simulink model "PM"  (R2018a)
settings: Solver=ode4  StartTime=0.0  StopTime=2  MaxStep=0.2  RelTol=1e-4
libraries: powerlib x20, simulink x13
settings Model: Creator=user  LastModifiedBy=user
settings CodeAppCC: StateflowObjectComments=on

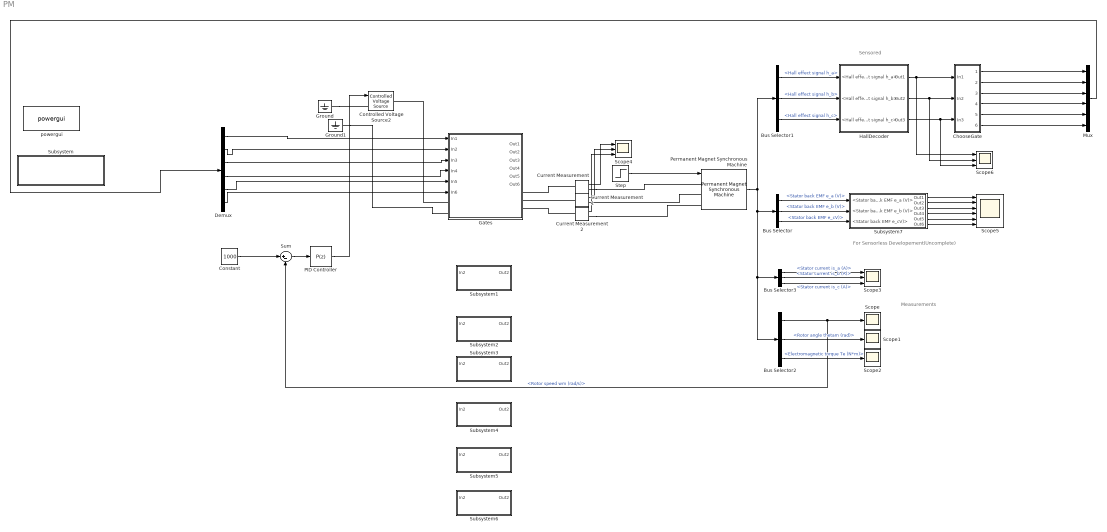
== system PM ==
  note: Measurements
  note: For Sensorless Developement(Uncomplete)
  note: Sensored
  Bus Selector : BusSelector  OutputSignals=Stator back EMF e_a (V),Stator back EMF e_b (V),Stator back EMF e_cV)
  Bus Selector1 : BusSelector  OutputSignals=Hall effect signal h_a,Hall effect signal h_b,Hall effect signal h_c
  Bus Selector2 : BusSelector  OutputSignals=Rotor speed wm (rad/s),Rotor angle thetam (rad),Electromagnetic torque Te (N*m)
  Bus Selector3 : BusSelector  OutputSignals=Stator current is_a (A),Stator current is_b (A),Stator current is_c (A)
  ChooseGate : Subsystem
  Constant : Constant  Value=1000
  Controlled Voltage Source2 : powerlib/Electrical Sources/Controlled Voltage Source  Initialize=on  Source_Type=AC  Amplitude=50  Phase=0  Frequency=0  Measurements=None
  Current Measurement : powerlib/Measurements/Current Measurement  PhasorSimulation=off  OutputType=Complex  PSBequivalent=0
  Current Measurement1 : powerlib/Measurements/Current Measurement  PhasorSimulation=off  OutputType=Complex  PSBequivalent=0
  Current Measurement2 : powerlib/Measurements/Current Measurement  PhasorSimulation=off  OutputType=Complex  PSBequivalent=0
  Demux : Demux  Outputs=6
  Gates : Subsystem
  Ground : powerlib/Elements/Ground  LConnTagsString=a
  Ground1 : powerlib/Elements/Ground  LConnTagsString=a
  HallDecoder : Subsystem
  Mux : Mux  Inputs=6
  PID Controller : simulink/Continuous/PID Controller  Controller=P  TimeDomain=Discrete-time  SampleTime=-1  IntegratorMethod=Forward Euler  FilterMethod=Forward Euler  Form=Parallel  UseFilter=on  ControllerParametersSource=internal  P=15.2669895958737  I=1  D=0  N=100  InitialConditionSource=internal  InitialConditionForIntegrator=0  InitialConditionForFilter=0  ExternalReset=none  LimitOutput=off  UpperSaturationLimit=inf  LowerSaturationLimit=-inf  LinearizeAsGain=on  AntiWindupMode=none  Kb=1  TrackingMode=off  Kt=1  PParamMin=[]  PParamMax=[]  IParamMin=[]  IParamMax=[]  DParamMin=[]  DParamMax=[]  NParamMin=[]  NParamMax=[]  KbParamMin=[]  KbParamMax=[]  KtParamMin=[]  KtParamMax=[]  POutMin=[]  POutMax=[]  IOutMin=[]  IOutMax=[]  DOutMin=[]  DOutMax=[]  NOutMin=[]  NOutMax=[]  KbOutMin=[]  KbOutMax=[]  KtOutMin=[]  KtOutMax=[]  IntegratorOutMin=[]  IntegratorOutMax=[]  FilterOutMin=[]  FilterOutMax=[]  SumOutMin=[]  SumOutMax=[]  SumI1OutMin=[]  SumI1OutMax=[]  SumI2OutMin=[]  SumI2OutMax=[]  SumI3OutMin=[]  SumI3OutMax=[]  SumDOutMin=[]  SumDOutMax=[]  SaturationOutMin=[]  SaturationOutMax=[]  IntegratorContinuousStateAttributes=''  IntegratorStateMustResolveToSignalObject=off  IntegratorRTWStateStorageClass=Auto  FilterContinuousStateAttributes=''  FilterStateMustResolveToSignalObject=off  FilterRTWStateStorageClass=Auto  DifferentiatorICPrevScaledInput=0  DifferentiatorOutMin=[]  DifferentiatorOutMax=[]  FilterDiffOutCoefMin=[]  FilterDiffOutCoefMax=[]  SumDenOutMin=[]  SumDenOutMax=[]  SumNumOutMin=[]  SumNumOutMax=[]  ReciprocalOutMin=[]  ReciprocalOutMax=[]  DivideOutMin=[]  DivideOutMax=[]  TunerSelectOption=Transfer Function Based (PID Tuner App)
  Permanent Magnet Synchronous Machine : powerlib/Machines/Permanent Magnet Synchronous Machine  NbPhases=3  FluxDistribution=Trapezoidal  RotorType=Round  MechanicalLoad=Torque Tm  PresetModel=No  ShowDetailedParameters=on  MeasurementBus=off  Resistance=2.8750  Inductance=8.5e-3  dqInductances=[8.5e-3, 8.5e-3]  La=0.000835  MachineConstant=Flux linkage established by magnets (V.s)  Flux=0.175  VoltageCst=146.6077  TorqueCst=1.4  Flat=120  Mechanical=[ 0.8e-3, 1e-3 4]  PolePairs=4  InitialConditions=[0,0, 0,0]  InitialConditions5ph=[0 0 0 0 0 0]  TsPowergui=0  TsBlock=-1  RefAngle=90 degrees behind phase A axis (modified Park)
      settings: SourceProductName=Simscape Power Systems
  Scope : Scope
  Scope1 : Scope
  Scope2 : Scope
  Scope3 : Scope  NumInputPorts=3
  Scope4 : Scope  NumInputPorts=3
  Scope5 : Scope  NumInputPorts=6
  Scope6 : Scope  NumInputPorts=3
  Step : Step  Time=0.01  After=2  SampleTime=0
  Subsystem : Subsystem
      settings: OpenFcn=open_system('power_new_palette')
      mask Display: disp(sprintf('Open Simscape Power Systems\n(Specialized Technology)\nPalette Library'));
  Subsystem1 : Subsystem
  Subsystem2 : Subsystem
  Subsystem3 : Subsystem
  Subsystem4 : Subsystem
  Subsystem5 : Subsystem
  Subsystem6 : Subsystem
  Subsystem7 : Subsystem
  Sum : Sum  Inputs=|+-
  powergui : powerlib/powergui  Priority=1  SimulationMode=Discrete  SampleTime=5e-6  frequency=60  Iterations=50  frequencyindice=0  Pbase=100e6  ErrMax=1e-4  UnitsV=kV  UnitsW=MW  buscounter=0  FunctionMessages=off  echomessages=off  EnableUseOfTLC=off  CurrentSourceSwitches=off  DisableSnubberDevices=off  DisableRonSwitches=off  DisableVfSwitches=off  DisplayEquations=off  SolverType=Tustin/Backward Euler (TBE)  Interpol=off  ExternalGateDelay=off  methode=off  Ts=100  x0status=blocks  SPID=on  SwTol=0  HookPort=off  RestoreLinks=warning  ResistiveCurrentMeasurement=off  Frange=[0:2:500]  Ylog=off  Xlog=on  ShowGrid=off  save=off  variable=ZData  structure=0  ZoomFFT=off  StartTime=0.0  cycles=1  DisplayStyle=1  fundamental=60  FreqAxis=off  MaxFrequency=1000  frequencyindicesteady=1  RmsSteady=1  display=off
  wires:
  Permanent Magnet Synchronous Machine/1 -> Bus Selector2/1, Bus Selector3/1, Bus Selector/1, Bus Selector1/1
  Bus Selector1/1 -> HallDecoder/1(<Hall effect signal h_a>)  "<Hall effect signal h_a>"
  Bus Selector1/2 -> HallDecoder/2(<Hall effect signal h_b>)  "<Hall effect signal h_b>"
  Bus Selector1/3 -> HallDecoder/3(<Hall effect signal h_c>)  "<Hall effect signal h_c>"
  HallDecoder/3(Out3) -> Scope6/3, ChooseGate/3(In3)
  HallDecoder/2(Out2) -> Scope6/2, ChooseGate/2(In2)
  HallDecoder/1(Out1) -> Scope6/1, ChooseGate/1(In1)
  Mux/1 -> Demux/1
  Bus Selector2/1 -> Sum/2, Scope/1  "<Rotor speed wm (rad/s)>"
  Bus Selector2/2 -> Scope1/1  "<Rotor angle thetam (rad)>"
  Bus Selector2/3 -> Scope2/1  "<Electromagnetic torque Te (N*m)>"
  Bus Selector3/2 -> Scope3/2  "<Stator current is_b (A)>"
  Bus Selector3/3 -> Scope3/3  "<Stator current is_c (A)>"
  Bus Selector3/1 -> Scope3/1  "<Stator current is_a (A)>"
  Current Measurement/1 -> Scope4/1
  Current Measurement2/1 -> Scope4/3
  Step/1 -> Permanent Magnet Synchronous Machine/1
  Current Measurement1/1 -> Scope4/2
  ChooseGate/1(Out1) -> Mux/1
  ChooseGate/2(Out2) -> Mux/2
  ChooseGate/3(Out3) -> Mux/3
  ChooseGate/4(Out4) -> Mux/4
  ChooseGate/5(Out5) -> Mux/5
  ChooseGate/6(Out6) -> Mux/6
  Bus Selector/1 -> Subsystem7/1(<Stator back EMF e_a (V)>)  "<Stator back EMF e_a (V)>"
  Bus Selector/2 -> Subsystem7/2(<Stator back EMF e_b (V)>)  "<Stator back EMF e_b (V)>"
  Bus Selector/3 -> Subsystem7/3(<Stator back EMF e_cV)>)  "<Stator back EMF e_cV)>"
  Subsystem7/1(Out1) -> Scope5/1
  Subsystem7/2(Out2) -> Scope5/2
  Subsystem7/3(Out3) -> Scope5/3
  Subsystem7/4(Out4) -> Scope5/4
  Subsystem7/5(Out5) -> Scope5/5
  Subsystem7/6(Out6) -> Scope5/6
  Demux/1 -> Gates/1(In1)
  Demux/2 -> Gates/2(In2)
  Demux/3 -> Gates/3(In3)
  Demux/4 -> Gates/4(In4)
  Demux/5 -> Gates/5(In5)
  Demux/6 -> Gates/6(In6)
  PID Controller/1 -> Controlled Voltage Source2/1
  Constant/1 -> Sum/1
  Sum/1 -> PID Controller/1
  connections:
  Ground/LConn1 -- Controlled Voltage Source2/LConn1
  Current Measurement/RConn1 -- Permanent Magnet Synchronous Machine/LConn1
  Permanent Magnet Synchronous Machine/LConn2 -- Current Measurement1/RConn1
  Current Measurement2/RConn1 -- Permanent Magnet Synchronous Machine/LConn3
  Current Measurement/LConn1 -- Gates/RConn1
  Gates/LConn1 -- Controlled Voltage Source2/RConn1
  Current Measurement1/LConn1 -- Gates/RConn2
  Ground1/LConn1 -- Gates/LConn2
  Current Measurement2/LConn1 -- Gates/RConn3

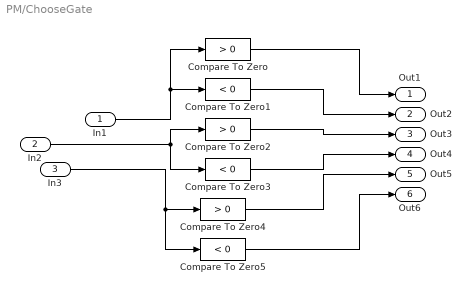
== system PM/ChooseGate ==
  In1 : Inport
  In2 : Inport  Port=2
  In3 : Inport  Port=3
  Compare To Zero : simulink/Logic and Bit Operations/Compare To Zero  relop=>  OutDataTypeStr=boolean  ZeroCross=off
  Compare To Zero1 : simulink/Logic and Bit Operations/Compare To Zero  relop=<  OutDataTypeStr=boolean  ZeroCross=off
  Compare To Zero2 : simulink/Logic and Bit Operations/Compare To Zero  relop=>  OutDataTypeStr=boolean  ZeroCross=off
  Compare To Zero3 : simulink/Logic and Bit Operations/Compare To Zero  relop=<  OutDataTypeStr=boolean  ZeroCross=off
  Compare To Zero4 : simulink/Logic and Bit Operations/Compare To Zero  relop=>  OutDataTypeStr=boolean  ZeroCross=off
  Compare To Zero5 : simulink/Logic and Bit Operations/Compare To Zero  relop=<  OutDataTypeStr=boolean  ZeroCross=off
  Out1 : Outport
  Out2 : Outport  Port=2
  Out3 : Outport  Port=3
  Out4 : Outport  Port=4
  Out5 : Outport  Port=5
  Out6 : Outport  Port=6
  wires:
  In3/1 -> Compare To Zero4/1, Compare To Zero5/1
  Compare To Zero/1 -> Out1/1
  In1/1 -> Compare To Zero/1, Compare To Zero1/1
  Compare To Zero1/1 -> Out2/1
  In2/1 -> Compare To Zero2/1, Compare To Zero3/1
  Compare To Zero5/1 -> Out6/1
  Compare To Zero4/1 -> Out5/1
  Compare To Zero3/1 -> Out4/1
  Compare To Zero2/1 -> Out3/1

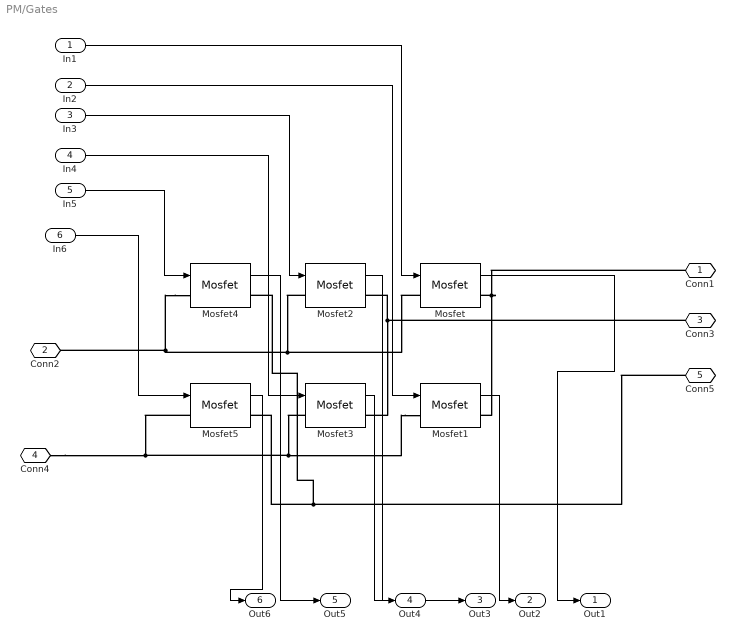
== system PM/Gates ==
  In1 : Inport
  In2 : Inport  Port=2
  In3 : Inport  Port=3
  In4 : Inport  Port=4
  In5 : Inport  Port=5
  In6 : Inport  Port=6
  Mosfet{,1..5} (6 alike) : powerlib/Power Electronics/Mosfet  Ron=0.1  Lon=0  Rd=0.01  Vfd=0  IC=0  Rs=1e5  Cs=inf  Measurements=on
  Conn1 : PMIOPort  Side=Right
  Conn2 : PMIOPort  Port=2  Side=Left
  Conn3 : PMIOPort  Port=3  Side=Right
  Conn4 : PMIOPort  Port=4  Side=Left
  Conn5 : PMIOPort  Port=5  Side=Right
  Out1 : Outport
  Out2 : Outport  Port=2
  Out3 : Outport  Port=3
  Out4 : Outport  Port=4
  Out5 : Outport  Port=5
  Out6 : Outport  Port=6
  wires:
  Mosfet/1 -> Out1/1
  In2/1 -> Mosfet1/1
  Mosfet1/1 -> Out2/1
  In3/1 -> Mosfet2/1
  Mosfet5/1 -> Out6/1
  In1/1 -> Mosfet/1
  Mosfet4/1 -> Out5/1
  Mosfet2/1 -> Out3/1
  Mosfet3/1 -> Out4/1
  In4/1 -> Mosfet3/1
  In5/1 -> Mosfet4/1
  In6/1 -> Mosfet5/1
  connections:
  Conn3/RConn1 -- Mosfet3/RConn1 -- Mosfet2/RConn1
  Conn5/RConn1 -- Mosfet4/RConn1 -- Mosfet5/RConn1
  Mosfet1/LConn1 -- Mosfet3/LConn1 -- Mosfet5/LConn1 -- Conn4/RConn1
  Mosfet4/LConn1 -- Mosfet2/LConn1 -- Mosfet/LConn1 -- Conn2/RConn1
  Mosfet/RConn1 -- Conn1/RConn1 -- Mosfet1/RConn1

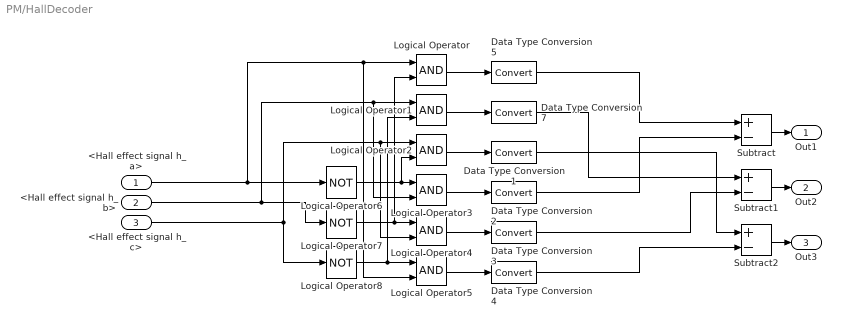
== system PM/HallDecoder ==
  <Hall effect signal h_a> : Inport
  <Hall effect signal h_b> : Inport  Port=2
  <Hall effect signal h_c> : Inport  Port=3
  Data Type Conversion{1..5,7} (6 alike) : DataTypeConversion
  Logical Operator{,1..5} (6 alike) : Logic  AllPortsSameDT=off  OutDataTypeStr=boolean
  Logical Operator6 : Logic  Operator=NOT  AllPortsSameDT=off  OutDataTypeStr=boolean
  Logical Operator7 : Logic  Operator=NOT  AllPortsSameDT=off  OutDataTypeStr=boolean
  Logical Operator8 : Logic  Operator=NOT  AllPortsSameDT=off  OutDataTypeStr=boolean
  Subtract : Sum  Inputs=+-
  Subtract1 : Sum  Inputs=+-
  Subtract2 : Sum  Inputs=+-
  Out1 : Outport
  Out2 : Outport  Port=2
  Out3 : Outport  Port=3
  wires:
  <Hall effect signal h_a>/1 -> Logical Operator6/1, Logical Operator5/2, Logical Operator/1
  Logical Operator6/1 -> Logical Operator2/2, Logical Operator3/1
  <Hall effect signal h_b>/1 -> Logical Operator7/1, Logical Operator1/1, Logical Operator3/2
  <Hall effect signal h_c>/1 -> Logical Operator8/1, Logical Operator4/2, Logical Operator2/1
  Logical Operator8/1 -> Logical Operator1/2, Logical Operator5/1
  Logical Operator7/1 -> Logical Operator4/1, Logical Operator/2
  Subtract2/1 -> Out3/1
  Subtract1/1 -> Out2/1
  Subtract/1 -> Out1/1
  Logical Operator/1 -> Data Type Conversion5/1
  Logical Operator1/1 -> Data Type Conversion7/1
  Logical Operator2/1 -> Data Type Conversion1/1
  Logical Operator3/1 -> Data Type Conversion2/1
  Logical Operator4/1 -> Data Type Conversion3/1
  Logical Operator5/1 -> Data Type Conversion4/1
  Data Type Conversion5/1 -> Subtract/1
  Data Type Conversion2/1 -> Subtract/2
  Data Type Conversion7/1 -> Subtract1/1
  Data Type Conversion3/1 -> Subtract1/2
  Data Type Conversion1/1 -> Subtract2/1
  Data Type Conversion4/1 -> Subtract2/2

== system PM/Subsystem ==

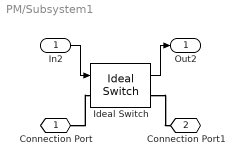
== system PM/Subsystem1 ==
  In2 : Inport
  Ideal Switch : powerlib/Power Electronics/Ideal Switch  Ron=0.001  Lon=0  IC=1  Rs=1e5  Cs=inf  Measurements=on
  Connection Port : PMIOPort  Side=Left
  Connection Port1 : PMIOPort  Port=2  Side=Right
  Out2 : Outport
  wires:
  In2/1 -> Ideal Switch/1
  Ideal Switch/1 -> Out2/1
  connections:
  Ideal Switch/RConn1 -- Connection Port1/RConn1
  Connection Port/RConn1 -- Ideal Switch/LConn1

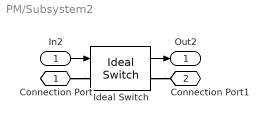
== system PM/Subsystem2 ==
  In2 : Inport
  Ideal Switch : powerlib/Power Electronics/Ideal Switch  Ron=0.001  Lon=0  IC=1  Rs=1e5  Cs=inf  Measurements=on
  Connection Port : PMIOPort  Side=Left
  Connection Port1 : PMIOPort  Port=2  Side=Right
  Out2 : Outport
  wires:
  In2/1 -> Ideal Switch/1
  Ideal Switch/1 -> Out2/1
  connections:
  Ideal Switch/RConn1 -- Connection Port1/RConn1
  Connection Port/RConn1 -- Ideal Switch/LConn1

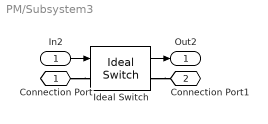
== system PM/Subsystem3 ==
  In2 : Inport
  Ideal Switch : powerlib/Power Electronics/Ideal Switch  Ron=0.001  Lon=0  IC=1  Rs=1e5  Cs=inf  Measurements=on
  Connection Port : PMIOPort  Side=Left
  Connection Port1 : PMIOPort  Port=2  Side=Right
  Out2 : Outport
  wires:
  In2/1 -> Ideal Switch/1
  Ideal Switch/1 -> Out2/1
  connections:
  Ideal Switch/RConn1 -- Connection Port1/RConn1
  Connection Port/RConn1 -- Ideal Switch/LConn1

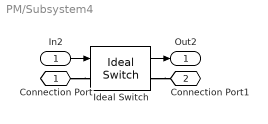
== system PM/Subsystem4 ==
  In2 : Inport
  Ideal Switch : powerlib/Power Electronics/Ideal Switch  Ron=0.001  Lon=0  IC=1  Rs=1e5  Cs=inf  Measurements=on
  Connection Port : PMIOPort  Side=Left
  Connection Port1 : PMIOPort  Port=2  Side=Right
  Out2 : Outport
  wires:
  In2/1 -> Ideal Switch/1
  Ideal Switch/1 -> Out2/1
  connections:
  Ideal Switch/RConn1 -- Connection Port1/RConn1
  Connection Port/RConn1 -- Ideal Switch/LConn1

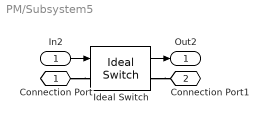
== system PM/Subsystem5 ==
  In2 : Inport
  Ideal Switch : powerlib/Power Electronics/Ideal Switch  Ron=0.001  Lon=0  IC=1  Rs=1e5  Cs=inf  Measurements=on
  Connection Port : PMIOPort  Side=Left
  Connection Port1 : PMIOPort  Port=2  Side=Right
  Out2 : Outport
  wires:
  In2/1 -> Ideal Switch/1
  Ideal Switch/1 -> Out2/1
  connections:
  Ideal Switch/RConn1 -- Connection Port1/RConn1
  Connection Port/RConn1 -- Ideal Switch/LConn1

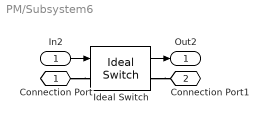
== system PM/Subsystem6 ==
  In2 : Inport
  Ideal Switch : powerlib/Power Electronics/Ideal Switch  Ron=0.001  Lon=0  IC=1  Rs=1e5  Cs=inf  Measurements=on
  Connection Port : PMIOPort  Side=Left
  Connection Port1 : PMIOPort  Port=2  Side=Right
  Out2 : Outport
  wires:
  In2/1 -> Ideal Switch/1
  Ideal Switch/1 -> Out2/1
  connections:
  Ideal Switch/RConn1 -- Connection Port1/RConn1
  Connection Port/RConn1 -- Ideal Switch/LConn1

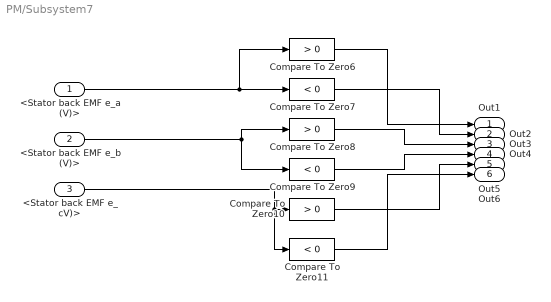
== system PM/Subsystem7 ==
  <Stator back EMF e_a (V)> : Inport
  <Stator back EMF e_b (V)> : Inport  Port=2
  <Stator back EMF e_cV)> : Inport  Port=3
  Compare To Zero10 : simulink/Logic and Bit Operations/Compare To Zero  relop=>  OutDataTypeStr=boolean  ZeroCross=off
  Compare To Zero11 : simulink/Logic and Bit Operations/Compare To Zero  relop=<  OutDataTypeStr=boolean  ZeroCross=off
  Compare To Zero6 : simulink/Logic and Bit Operations/Compare To Zero  relop=>  OutDataTypeStr=boolean  ZeroCross=off
  Compare To Zero7 : simulink/Logic and Bit Operations/Compare To Zero  relop=<  OutDataTypeStr=boolean  ZeroCross=off
  Compare To Zero8 : simulink/Logic and Bit Operations/Compare To Zero  relop=>  OutDataTypeStr=boolean  ZeroCross=off
  Compare To Zero9 : simulink/Logic and Bit Operations/Compare To Zero  relop=<  OutDataTypeStr=boolean  ZeroCross=off
  Out1 : Outport
  Out2 : Outport  Port=2
  Out3 : Outport  Port=3
  Out4 : Outport  Port=4
  Out5 : Outport  Port=5
  Out6 : Outport  Port=6
  wires:
  <Stator back EMF e_cV)>/1 -> Compare To Zero11/1, Compare To Zero10/1
  Compare To Zero8/1 -> Out3/1
  Compare To Zero9/1 -> Out4/1
  Compare To Zero11/1 -> Out6/1
  <Stator back EMF e_b (V)>/1 -> Compare To Zero9/1, Compare To Zero8/1
  Compare To Zero6/1 -> Out1/1
  <Stator back EMF e_a (V)>/1 -> Compare To Zero7/1, Compare To Zero6/1
  Compare To Zero7/1 -> Out2/1
  Compare To Zero10/1 -> Out5/1
